simulink model "sim_mixed"  (R2020b)
settings: Solver=VariableStepAuto  StartTime=0.0  StopTime=300  RelTol=1e-3
values from neighbouring files (symbols this model uses):
  L10 = 10    [quad_tank_setup.m]
  L20 = 14    [quad_tank_setup.m]
  L30 = ((1-gamma2)*Kp*Vp20/Ao3)^2/(2*g)    [quad_tank_setup.m]
  L40 = ((1-gamma1)*Kp*Vp10/Ao4)^2/(2*g)    [quad_tank_setup.m]
  plant_discrete = c2d(plant,Ts)    [main_EMPC_QuadTank.m]
  Vp10 = Ao1*sqrt(2*g*L10)/(gamma1*Kp)-(1-gamma2)*Vp20/gamma1    [quad_tank_setup.m]
  Vp20 = Ao1*(1-gamma1)*sqrt(2*g*L10)/(((1-gamma1)*(1-gamma2)-gamma1*gamma2)*Kp)-Ao2*(gamma1)*sqrt(2*g*L20)/(((1-gamma1)*(1-gamma2)-gamma1*gamma2)*Kp)    [quad_tank_setup.m]
libraries: mpclib x2
settings Model: Creator=andrewralea  LastModifiedBy=andrewralea
settings ConfigComp: PLC_TargetIDE=twincat3

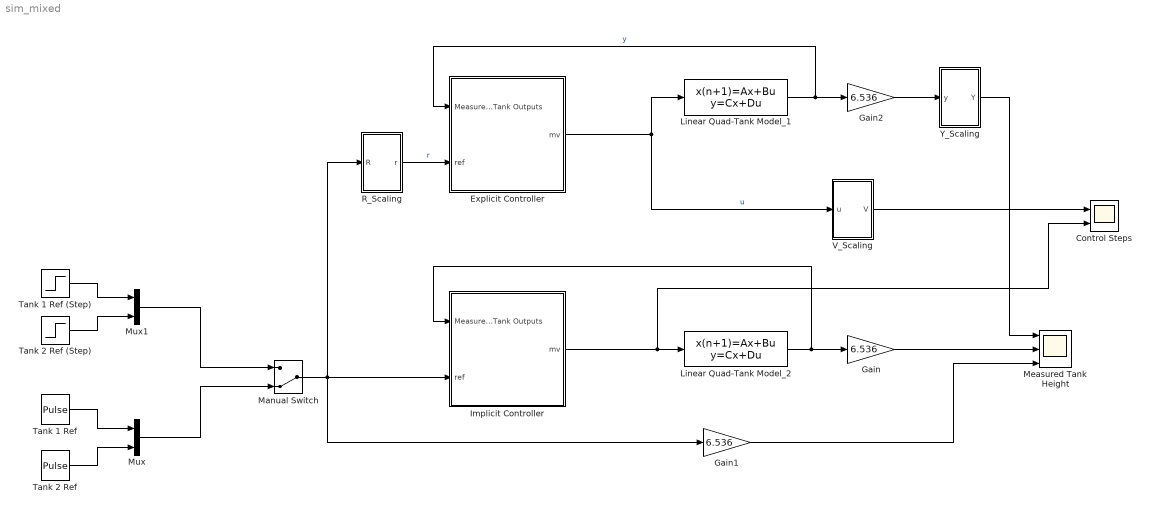
== system sim_mixed ==
  Control Steps : Scope  NumInputPorts=2
  Explicit Controller : Subsystem  TreatAsAtomicUnit=on
  Gain : Gain  Gain=6.536
  Gain1 : Gain  Gain=6.536
  Gain2 : Gain  Gain=6.536
  Implicit Controller : Subsystem  TreatAsAtomicUnit=on
  Linear Quad-Tank Model_1 : DiscreteStateSpace  A=plant_discrete.A  B=plant_discrete.B  C=plant_discrete.C  D=plant_discrete.D  SampleTime=-1
  Linear Quad-Tank Model_2 : DiscreteStateSpace  A=plant_discrete.A  B=plant_discrete.B  C=plant_discrete.C  D=plant_discrete.D  InitialCondition=[L10, L20, L30, L40]  SampleTime=-1
  Manual Switch : ManualSwitch  CurrentSetting=0
  Measured Tank Height : Scope  NumInputPorts=3
  Mux : Mux  Inputs=2
  Mux1 : Mux  Inputs=2
  R_Scaling : Subsystem
  Tank 1 Ref : DiscretePulseGenerator  PulseType=Time based  Amplitude=L10 / 6.536  Period=100  PulseWidth=50
  Tank 1 Ref (Step) : Step  Time=100  Before=L10 / 6.536  After=2.5  SampleTime=0
  Tank 2 Ref : DiscretePulseGenerator  PulseType=Time based  Amplitude=L20 / 6.536  Period=200  PulseWidth=50
  Tank 2 Ref (Step) : Step  Time=100  Before=L20 / 6.536  After=3  SampleTime=0
  V_Scaling : Subsystem
  Y_Scaling : Subsystem
  wires:
  Linear Quad-Tank Model_2/1 -> Implicit Controller/1(Measured Tank Outputs), Gain/1
  Gain/1 -> Measured Tank Height/2
  Gain1/1 -> Measured Tank Height/3
  Tank 1 Ref/1 -> Mux/1
  Tank 2 Ref/1 -> Mux/2
  Gain2/1 -> Y_Scaling/1(y)
  Tank 2 Ref (Step)/1 -> Mux1/2
  Tank 1 Ref (Step)/1 -> Mux1/1
  Mux1/1 -> Manual Switch/1
  Manual Switch/1 -> R_Scaling/1(R), Implicit Controller/2(ref), Gain1/1
  R_Scaling/1(r) -> Explicit Controller/2(ref)  "r"
  Linear Quad-Tank Model_1/1 -> Explicit Controller/1(Measured Tank Outputs), Gain2/1  "y"
  Mux/1 -> Manual Switch/2
  Explicit Controller/1(mv) -> Linear Quad-Tank Model_1/1, V_Scaling/1(u)  "u"
  Y_Scaling/1(Y) -> Measured Tank Height/1
  V_Scaling/1(V) -> Control Steps/1
  Implicit Controller/1(mv) -> Control Steps/2, Linear Quad-Tank Model_2/1

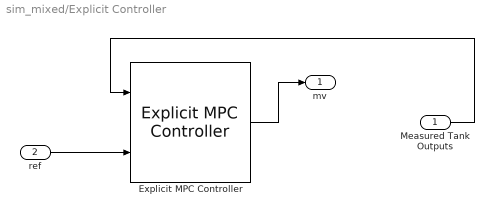
== system sim_mixed/Explicit Controller ==
  Measured Tank Outputs : Inport
  ref : Inport  Port=2
  Explicit MPC Controller : mpclib/Explicit MPC Controller  SCDEnableBlockLinearizationSpecification=on  empcobj=mpcobjExplicitSimplified  is_multiple=0  enable_value=0  return_u0=off  md_inport=off  mv_inport=off  return_status=off  return_region=off  return_state=off  state_inport=off  BlockDataType=double  SampleTimeInherited=off  switch_inport=off
      settings: SourceProductBaseCode=MP
  mv : Outport
  wires:
  ref/1 -> Explicit MPC Controller/2
  Measured Tank Outputs/1 -> Explicit MPC Controller/1
  Explicit MPC Controller/1 -> mv/1

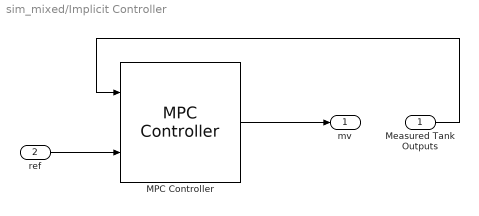
== system sim_mixed/Implicit Controller ==
  Measured Tank Outputs : Inport
  ref : Inport  Port=2
  MPC Controller : mpclib/MPC Controller  SCDEnableBlockLinearizationSpecification=on  mpcobj=mpcobj  is_multiple=0  enable_value=0  return_u0=off  updateMPCinCallerWorkspace=on  md_inport=off  mv_inport=off  uref_inport=off  return_cost=off  return_mvseq=off  return_qpstatus=off  return_xseq=off  return_state=off  return_ovseq=off  state_inport=off  umin_inport=off  umax_inport=off  ymin_inport=off  ymax_inport=off  cc_inport=off  ywt_inport=off  uwt_inport=off  duwt_inport=off  rhoeps_inport=off  pm_inport=off  MaximumP=10  HorizonChoice=FixedHorizon  n_ts=0.1  n_p=6  n_mv=2  n_md=0  n_ud=0  n_mo=2  n_uo=0  BlockDataType=double  SampleTimeInherited=off  switch_inport=off
  mv : Outport
  wires:
  Measured Tank Outputs/1 -> MPC Controller/1
  ref/1 -> MPC Controller/2
  MPC Controller/1 -> mv/1

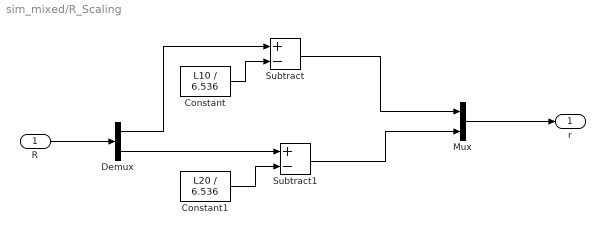
== system sim_mixed/R_Scaling ==
  R : Inport
  Constant : Constant  Value=L10 / 6.536
  Constant1 : Constant  Value=L20 / 6.536
  Demux : Demux  Outputs=2
  Mux : Mux  Inputs=2
  Subtract : Sum  Inputs=+-
  Subtract1 : Sum  Inputs=+-
  r : Outport
  wires:
  R/1 -> Demux/1
  Demux/1 -> Subtract/1
  Constant/1 -> Subtract/2
  Constant1/1 -> Subtract1/2
  Demux/2 -> Subtract1/1
  Subtract/1 -> Mux/1
  Subtract1/1 -> Mux/2
  Mux/1 -> r/1

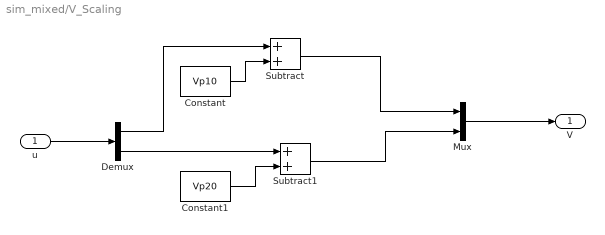
== system sim_mixed/V_Scaling ==
  u : Inport
  Constant : Constant  Value=Vp10
  Constant1 : Constant  Value=Vp20
  Demux : Demux  Outputs=2
  Mux : Mux  Inputs=2
  Subtract : Sum
  Subtract1 : Sum
  V : Outport
  wires:
  u/1 -> Demux/1
  Demux/1 -> Subtract/1
  Constant/1 -> Subtract/2
  Constant1/1 -> Subtract1/2
  Demux/2 -> Subtract1/1
  Subtract/1 -> Mux/1
  Subtract1/1 -> Mux/2
  Mux/1 -> V/1

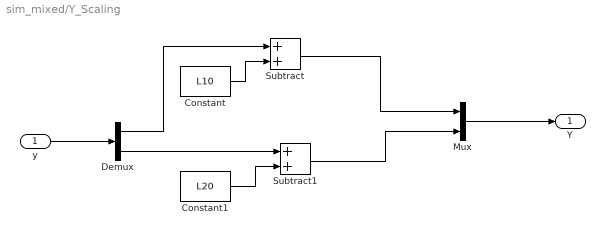
== system sim_mixed/Y_Scaling ==
  y : Inport
  Constant : Constant  Value=L10
  Constant1 : Constant  Value=L20
  Demux : Demux  Outputs=2
  Mux : Mux  Inputs=2
  Subtract : Sum
  Subtract1 : Sum
  Y : Outport
  wires:
  y/1 -> Demux/1
  Demux/1 -> Subtract/1
  Constant/1 -> Subtract/2
  Constant1/1 -> Subtract1/2
  Demux/2 -> Subtract1/1
  Subtract/1 -> Mux/1
  Subtract1/1 -> Mux/2
  Mux/1 -> Y/1
